simulink model "mpcHighway"  (R2025a)
settings: Solver=VariableStepAuto  StartTime=0.0  StopTime=inf  FixedStep=0.001  RelTol=1e-3
PreLoadFcn:
  | setUpModel
model workspace (MAT data in the model file):
  firstWarning = 0
  originalScenarioChecksum = 'F73A6DA3C723D3CA73A6F931B7A52A9C'
values from neighbouring files (symbols this model uses):
  accel_vec = (-4:0.5:4)'    [setUpModel.m]
  C = [C1 zeros(1,2); zeros(2,2) C2]    [setUpModel.m]    (also in vehicle_grey_model.m = [1, 0, 0, 0)
  curvature = (DX.*D2Y - DY.*D2X) ./(DX.^2+DY.^2).^(3/2)    [setUpModel.m]
  D = [D1 zeros(1,1); zeros(2,1) D2]    [setUpModel.m]    (also in vehicle_grey_model.m = zeros(3, 2))
  gradbp = linspace(0,totalDistance,100)    [setUpModel.m]
  psi_o = 0*(pi/180)    (= 0)    [setUpModel.m]
  psi_path = unwrap(psi_path)    [setUpModel.m]
  s = size(xRef)    [setUpModel.m]
  vel = lookUpt(2:42,2:31)*4/5    [setUpModel.m]
  vel_vec = 0:2:20    [setUpModel.m]
  X_o = xRef(1)    [setUpModel.m]
  xlt = lookUpt(2:42,1)    [setUpModel.m]
  xRef2 = interp1(distbp,xRef,gradbp,'pchip')    [setUpModel.m]
  xRef2s = smooth(gradbp,xRef2)    [setUpModel.m]
  Y_o = yRef(1)    [setUpModel.m]
  ylt = lookUpt(1,2:31)    [setUpModel.m]
  yRef2 = interp1(distbp,yRef,gradbp,'pchip')    [setUpModel.m]
  yRef2s = smooth(gradbp,yRef2)    [setUpModel.m]
undefined symbols (not defined in the file or in its folder): deg, rad
libraries: vehdynlibtirecommon x4, autolibutils x3, vehdynlibviscommon x1, aerolibconvert2 x1, simulink_extras x1, drivingscenarioandsensors x1, mpcadaslib x1, vehdynlibtire x1, sim3dlib x1, sim3dautolib x1, autolibshared x1
(part 2 of 2)

== matlab function mpcHighway/Final Trajectory Bird's-Eye Visualization/MATLAB Function ==
  data: pos input; egoActor output Bus: BusActorsActors; vel input; yaw input; yawRate input
function egoActor = packEgo(pos,vel,yaw,yawRate)
% Pack ego information into a single ego actor bus
%
% Imoprtant note:
% Output is a bus of type BusActorsActors. This is the same bus used by the
% Scenario Reader to output an individual actor. If you change the
% output bus name of Scenario Reader, change the output bus name here
% as well by clicking on 'Edit Data' in the menu above.

egoActor = struct(...
    'ActorID',46,...
    'Position', [pos(1) pos(2) 0], ...
    'Velocity', [vel(1) vel(2) 0], ...
    'Roll', 0, ...
    'Pitch', 0, ...
    'Yaw', yaw, ...
    'AngularVelocity', [0 0 yawRate]);
